simulink model "Fig235"  (R2014a)
settings: Solver=ode3  StartTime=0.0  StopTime=100  FixedStep=2e-5  RelTol=1e-5
libraries: dspstat3 x4, commfilt2 x1, commchan3 x1
settings Model: Creator=Dennis Silage  LastModifiedBy=Silage
settings SolverCC: AutoInsertRateTranBlk=on
settings DataIOCC: SignalLoggingSaveFormat=ModelDataLogs
settings OptimizationCC: ExpressionDepthLimit=2147483647  InitFltsAndDblsToZero=on
settings DebuggingCC: UnderspecifiedInitializationDetection=Classic  SolverPrmCheckMsg=none  FcnCallInpInsideContextMsg=UseLocalSettings  StateNameClashWarn=warning
settings GRTTargetCC: CombineOutputUpdateFcns=off  GRTInterface=on

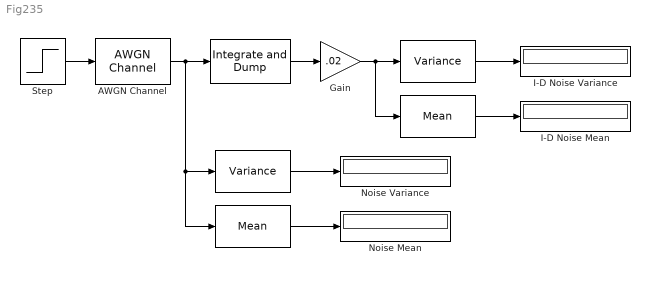
== system Fig235 ==
  " " : commfilt2/Integrate and Dump  obssamples=50  offsetsamples=0  nodump=on  roundingMode=Floor  overflowMode=off
  "   " : dspstat3/Variance  run=on  reset_popup=None  directionMode=Each column  dimension=1  treatSBRowAsCol=on  roiEnable=off  roiType=Rectangles  roiPortion=Entire ROI  roiOutput=Individual statistics for each ROI  roiFlag=off  roundingMode=Floor  overflowMode=off
  "    " : dspstat3/Mean  run=on  reset_popup=None  directionMode=Each column  dimension=1  treatSBRowAsCol=on  roiEnable=off  roiType=Rectangles  roiPortion=Entire ROI  roiOutput=Individual statistics for each ROI  roiFlag=off  outputDataTypeStr=Inherit: Same as accumulator  outputLastDataTypeStr=Inherit: Same as accumulator  outputMin=[]  outputMax=[]  roundingMode=Floor  overflowMode=off
  "      " : dspstat3/Variance  run=on  reset_popup=None  directionMode=Each column  dimension=1  treatSBRowAsCol=on  roiEnable=off  roiType=Rectangles  roiPortion=Entire ROI  roiOutput=Individual statistics for each ROI  roiFlag=off  roundingMode=Floor  overflowMode=off
  "       " : dspstat3/Mean  run=on  reset_popup=None  directionMode=Each column  dimension=1  treatSBRowAsCol=on  roiEnable=off  roiType=Rectangles  roiPortion=Entire ROI  roiOutput=Individual statistics for each ROI  roiFlag=off  outputDataTypeStr=Inherit: Same as accumulator  outputLastDataTypeStr=Inherit: Same as accumulator  outputMin=[]  outputMax=[]  roundingMode=Floor  overflowMode=off
  AWGN Channel : commchan3/AWGN Channel  InputProcessing=Inherited (this choice will be removed - see release notes)  seed=randseed  noiseMode=Variance from mask  EbNodB=10  EsNodB=10  SNRdB=10  bitsPerSym=1  Ps=1  Tsym=1  variance=10
  Gain : Gain  Gain=.02
  I-D Noise Mean : Display
  I-D Noise Variance : Display
  Noise Mean : Display
  Noise Variance : Display
  Step : Step  Time=0  After=0  SampleTime=2e-5
  wires:
  AWGN Channel/1 -> " "/1, "      "/1, "       "/1
  Step/1 -> AWGN Channel/1
  "      "/1 -> Noise Variance/1
  "       "/1 -> Noise Mean/1
  " "/1 -> Gain/1
  Gain/1 -> "   "/1, "    "/1
  "    "/1 -> I-D Noise Mean/1
  "   "/1 -> I-D Noise Variance/1
